simulink model "YawModel_R1"  (R2013a)
settings: Solver=ode45  StartTime=0.0  StopTime=10  RelTol=1e-3
values from neighbouring files (symbols this model uses):
  Kp_Yaw = 1.59458708377    [Yaw_Controller.mat]
  T_I = (1/(2*v))*((imag(DCL_Pole_1)/2)-(real(DCL_Pole_1)*v))    [Height_Controller_PID.m]
undefined symbols (not defined in the file or in its folder): D, I_Psi, J, Kw, Motor_TimeConstant, Speed_yIntercept
libraries: simulink x3
settings Model: Creator=Ross  LastModifiedBy=Ross

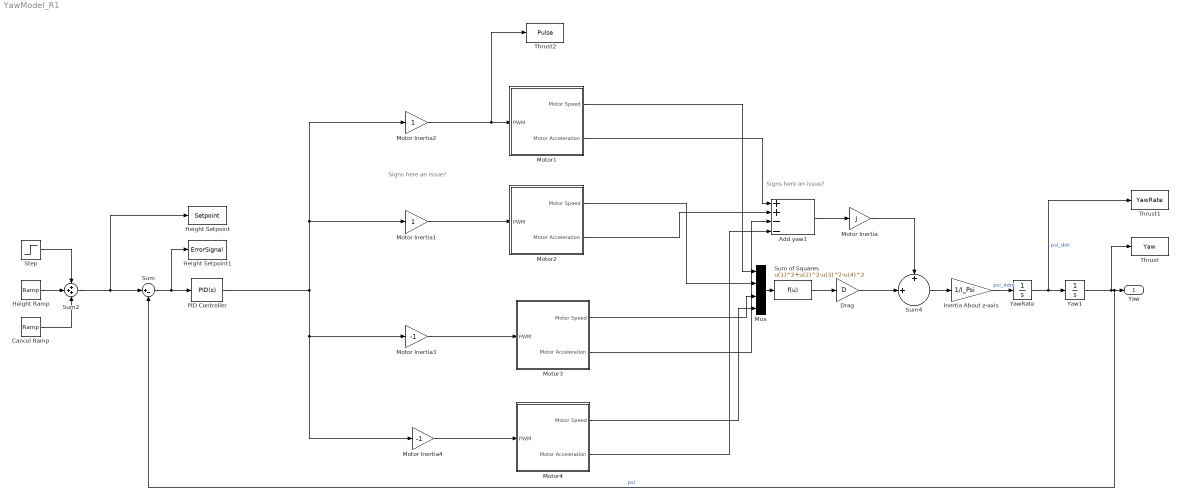
== system YawModel_R1 ==
  note: Signs here
      | an issue?
  note: Signs here
      | an issue?
  Add yaw1 : Sum  Inputs=++--
  Cancel Ramp : simulink/Sources/Ramp  slope=-1  start=2  X0=0
  Drag : Gain  Gain=D
  Height Ramp : simulink/Sources/Ramp  slope=1  start=1  X0=0
  Height Setpoint : ToWorkspace  VariableName=Setpoint  SampleTime=-1  SaveFormat=Timeseries
  Height Setpoint1 : ToWorkspace  VariableName=ErrorSignal  SampleTime=-1  SaveFormat=Timeseries
  Inertia About z-axis : Gain  Gain=1/I_Psi
  Motor Inertia : Gain  Gain=J
  Motor Inertia1 : Gain
  Motor Inertia2 : Gain
  Motor Inertia3 : Gain  Gain=-1
  Motor Inertia4 : Gain  Gain=-1
  Motor1 : Subsystem
  Motor2 : Subsystem
  Motor3 : Subsystem
  Motor4 : Subsystem
  Mux : Mux
  PID Controller : simulink/Continuous/PID Controller  Controller=PID  TimeDomain=Continuous-time  SampleTime=1  IntegratorMethod=Forward Euler  FilterMethod=Forward Euler  Form=Ideal  P=Kp_Yaw  I=1/T_I  D=T_I/4  N=100  InitialConditionSource=internal  InitialConditionForIntegrator=0  InitialConditionForFilter=0  ExternalReset=none  LimitOutput=off  UpperSaturationLimit=2  LowerSaturationLimit=0  LinearizeAsGain=on  AntiWindupMode=clamping  Kb=1  TrackingMode=off  Kt=1  PParamMin=[]  PParamMax=[]  IParamMin=[]  IParamMax=[]  DParamMin=[]  DParamMax=[]  NParamMin=[]  NParamMax=[]  KbParamMin=[]  KbParamMax=[]  KtParamMin=[]  KtParamMax=[]  POutMin=[]  POutMax=[]  IOutMin=[]  IOutMax=[]  DOutMin=[]  DOutMax=[]  NOutMin=[]  NOutMax=[]  KbOutMin=[]  KbOutMax=[]  KtOutMin=[]  KtOutMax=[]  IntegratorOutMin=[]  IntegratorOutMax=[]  FilterOutMin=[]  FilterOutMax=[]  SumOutMin=[]  SumOutMax=[]  SumI1OutMin=[]  SumI1OutMax=[]  SumI2OutMin=[]  SumI2OutMax=[]  SumI3OutMin=[]  SumI3OutMax=[]  SumDOutMin=[]  SumDOutMax=[]  SaturationOutMin=[]  SaturationOutMax=[]  IntegratorContinuousStateAttributes=''  IntegratorStateMustResolveToSignalObject=off  IntegratorRTWStateStorageClass=Auto  FilterContinuousStateAttributes=''  FilterStateMustResolveToSignalObject=off  FilterRTWStateStorageClass=Auto
  Step : Step  Time=2  After=2  SampleTime=0
  Sum : Sum  Inputs=|+-
  Sum of Squares : Fcn  Expr=u(1)^2+u(2)^2-u(3)^2-u(4)^2
  Sum2 : Sum  Inputs=+++
  Sum4 : Sum  Inputs=+|||+||||
  Thrust : ToWorkspace  VariableName=Yaw  SampleTime=-1  SaveFormat=Timeseries
  Thrust1 : ToWorkspace  VariableName=YawRate  SampleTime=-1  SaveFormat=Timeseries
  Thrust2 : ToWorkspace  VariableName=Pulse  SampleTime=-1  SaveFormat=Timeseries
  Yaw1 : Integrator  LowerSaturationLimit=0
  YawRate : Integrator
  Yaw : Outport
  wires:
  PID Controller/1 -> Motor Inertia4/1, Motor Inertia3/1, Motor Inertia1/1, Motor Inertia2/1
  Step/1 -> Sum2/1
  Height Ramp/1 -> Sum2/2
  Cancel Ramp/1 -> Sum2/3
  Sum2/1 -> Height Setpoint/1, Sum/1
  Sum/1 -> Height Setpoint1/1, PID Controller/1
  Add yaw1/1 -> Motor Inertia/1
  Motor Inertia/1 -> Sum4/1
  Sum of Squares/1 -> Drag/1
  Drag/1 -> Sum4/2
  Sum4/1 -> Inertia About z-axis/1
  Mux/1 -> Sum of Squares/1
  Motor1/1(Motor Speed) -> Mux/1
  Motor2/1(Motor Speed) -> Mux/2
  Motor3/1(Motor Speed) -> Mux/3
  Motor4/1(Motor Speed) -> Mux/4
  Motor1/2(Motor Acceleration) -> Add yaw1/1
  Motor2/2(Motor Acceleration) -> Add yaw1/2
  Motor3/2(Motor Acceleration) -> Add yaw1/3
  Motor4/2(Motor Acceleration) -> Add yaw1/4
  Motor Inertia2/1 -> Thrust2/1, Motor1/1(PWM)
  Motor Inertia1/1 -> Motor2/1(PWM)
  Motor Inertia3/1 -> Motor3/1(PWM)
  Motor Inertia4/1 -> Motor4/1(PWM)
  Yaw1/1 -> Thrust/1, Sum/2, Yaw/1  "psi"
  YawRate/1 -> Thrust1/1, Yaw1/1  "psi_dot"
  Inertia About z-axis/1 -> YawRate/1  "psi_ddot"

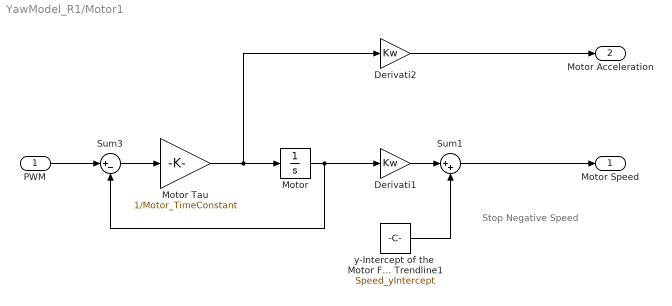
== system YawModel_R1/Motor1 ==
  note: Stop Negative
      | Speed
  PWM : Inport
  Derivati1 : Gain  Gain=Kw
  Derivati2 : Gain  Gain=Kw
  Motor : Integrator
  Motor Tau : Gain  Gain=1/Motor_TimeConstant
  Sum1 : Sum  Inputs=|++
  Sum3 : Sum  Inputs=|+-
  y-Intercept of the  Motor Forc Trendline1 : Constant  Value=Speed_yIntercept
  Motor Speed : Outport
  Motor Acceleration : Outport  Port=2
  wires:
  Motor Tau/1 -> Derivati2/1, Motor/1
  Motor/1 -> Derivati1/1, Sum3/2
  PWM/1 -> Sum3/1
  Sum3/1 -> Motor Tau/1
  y-Intercept of the  Motor Forc Trendline1/1 -> Sum1/2
  Derivati1/1 -> Sum1/1
  Sum1/1 -> Motor Speed/1
  Derivati2/1 -> Motor Acceleration/1

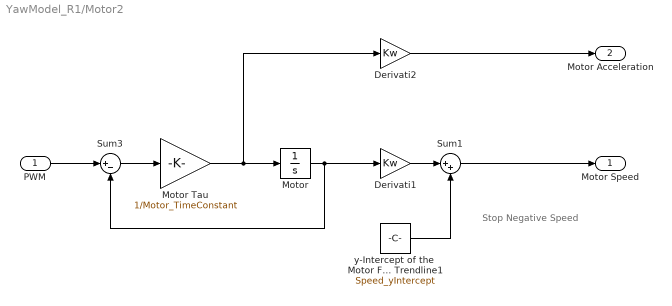
== system YawModel_R1/Motor2 ==
  note: Stop Negative
      | Speed
  PWM : Inport
  Derivati1 : Gain  Gain=Kw
  Derivati2 : Gain  Gain=Kw
  Motor : Integrator
  Motor Tau : Gain  Gain=1/Motor_TimeConstant
  Sum1 : Sum  Inputs=|++
  Sum3 : Sum  Inputs=|+-
  y-Intercept of the  Motor Forc Trendline1 : Constant  Value=Speed_yIntercept
  Motor Speed : Outport
  Motor Acceleration : Outport  Port=2
  wires:
  Motor Tau/1 -> Derivati2/1, Motor/1
  Motor/1 -> Derivati1/1, Sum3/2
  PWM/1 -> Sum3/1
  Sum3/1 -> Motor Tau/1
  y-Intercept of the  Motor Forc Trendline1/1 -> Sum1/2
  Derivati1/1 -> Sum1/1
  Sum1/1 -> Motor Speed/1
  Derivati2/1 -> Motor Acceleration/1

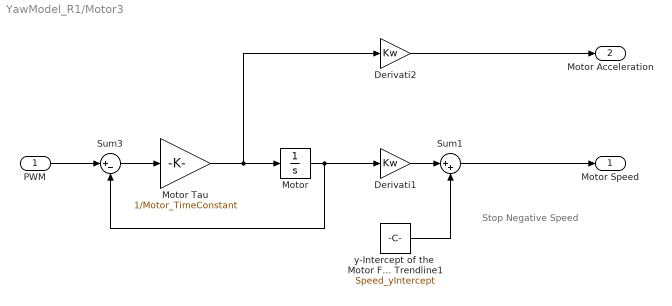
== system YawModel_R1/Motor3 ==
  note: Stop Negative
      | Speed
  PWM : Inport
  Derivati1 : Gain  Gain=Kw
  Derivati2 : Gain  Gain=Kw
  Motor : Integrator
  Motor Tau : Gain  Gain=1/Motor_TimeConstant
  Sum1 : Sum  Inputs=|++
  Sum3 : Sum  Inputs=|+-
  y-Intercept of the  Motor Forc Trendline1 : Constant  Value=Speed_yIntercept
  Motor Speed : Outport
  Motor Acceleration : Outport  Port=2
  wires:
  Motor Tau/1 -> Derivati2/1, Motor/1
  Motor/1 -> Derivati1/1, Sum3/2
  PWM/1 -> Sum3/1
  Sum3/1 -> Motor Tau/1
  y-Intercept of the  Motor Forc Trendline1/1 -> Sum1/2
  Derivati1/1 -> Sum1/1
  Sum1/1 -> Motor Speed/1
  Derivati2/1 -> Motor Acceleration/1

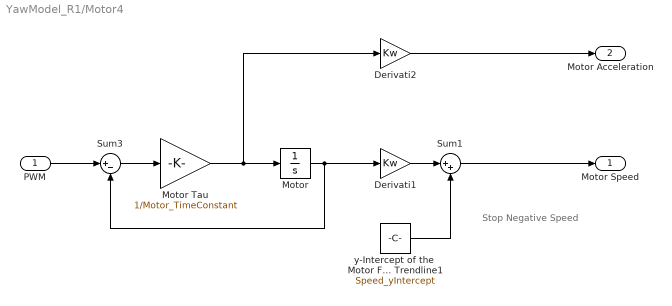
== system YawModel_R1/Motor4 ==
  note: Stop Negative
      | Speed
  PWM : Inport
  Derivati1 : Gain  Gain=Kw
  Derivati2 : Gain  Gain=Kw
  Motor : Integrator
  Motor Tau : Gain  Gain=1/Motor_TimeConstant
  Sum1 : Sum  Inputs=|++
  Sum3 : Sum  Inputs=|+-
  y-Intercept of the  Motor Forc Trendline1 : Constant  Value=Speed_yIntercept
  Motor Speed : Outport
  Motor Acceleration : Outport  Port=2
  wires:
  Motor Tau/1 -> Derivati2/1, Motor/1
  Motor/1 -> Derivati1/1, Sum3/2
  PWM/1 -> Sum3/1
  Sum3/1 -> Motor Tau/1
  y-Intercept of the  Motor Forc Trendline1/1 -> Sum1/2
  Derivati1/1 -> Sum1/1
  Sum1/1 -> Motor Speed/1
  Derivati2/1 -> Motor Acceleration/1
